simulink model "Simple_Pindulum"  (R2023a)
settings: Solver=VariableStepAuto  StartTime=0.0  StopTime=10  MaxStep=0.01  RelTol=1e-3
values from neighbouring files (symbols this model uses):
  L = L_Values(i)    [Simple_pendulum.m]
settings Model: Creator=Mohamed Ezzelrgal  LastModifiedBy=Mohamed Ezzelrgal

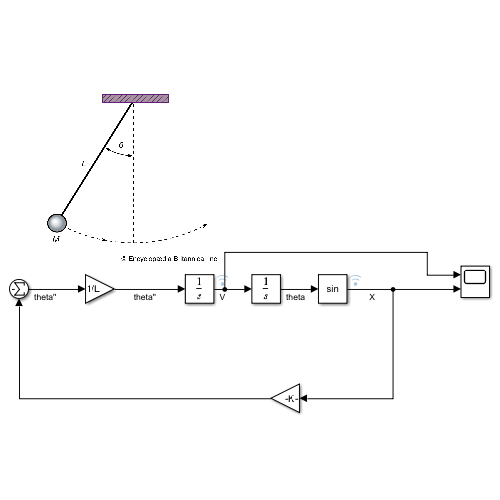
[thumbnail: Simulink's stored preview of the top-level diagram]
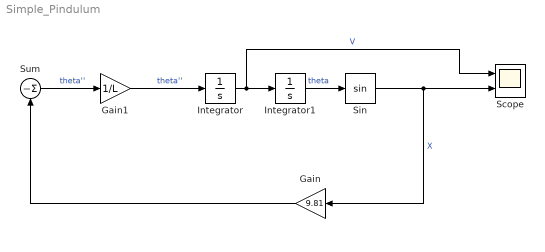
== system Simple_Pindulum ==
  Gain : Gain  Gain=9.81
  Gain1 : Gain  Gain=1/L
  Integrator : Integrator
  Integrator1 : Integrator  InitialCondition=1
  Scope : Scope  NumInputPorts=2
  Sin : Trigonometry
  Sum : Sum  Inputs=|-
  wires:
  Integrator/1 -> Scope/1, Integrator1/1  "V"
  Integrator1/1 -> Sin/1  "theta"
  Sin/1 -> Gain/1, Scope/2  "X"
  Gain1/1 -> Integrator/1  "theta''"
  Sum/1 -> Gain1/1  "theta''"
  Gain/1 -> Sum/1
